simulink model "kalman"  (R2021a)
settings: Solver=VariableStepAuto  StartTime=0.0  StopTime=10.0  RelTol=1e-3
values from neighbouring files (symbols this model uses):
  A = [0,0,1,0;0,0,0,1;0,(g*mp)/mc,-d1/mc,-d2/(L*mc);0,(g*(mc+mp))/(L*mc),-d1/(L*mc),-(d2*(mc+mp))/(L*L*mc*mp)]    [assgn_4.m]
  B = [0;0;1/mc;1/(L*mc)]    [assgn_4.m]
  C = [1,0,0,0]    [assgn_4.m]
undefined symbols (not defined in the file or in its folder): K1
libraries: simulink x1
settings Model: Creator=hp  LastModifiedBy=hp

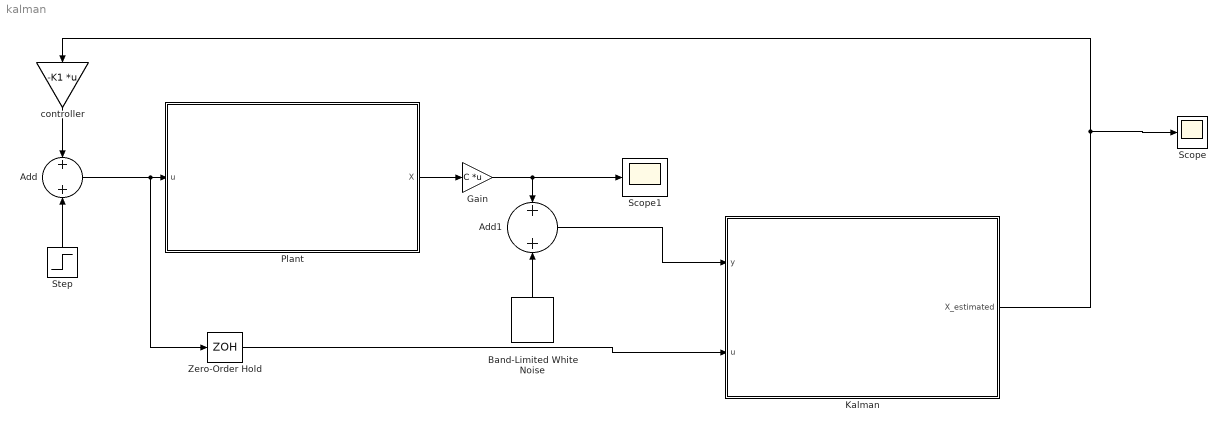
== system kalman ==
  Add : Sum
  Add1 : Sum
  Band-Limited White Noise : simulink/Sources/Band-Limited White Noise  Cov=[0.005]  Ts=0.1  seed=[23341]
  Gain : Gain  Gain=C  Multiplication=Matrix(K*u)
  Kalman : Subsystem
  Plant : Subsystem
  Scope : Scope
  Scope1 : Scope
  Step : Step  Time=0  SampleTime=0
  Zero-Order Hold : ZeroOrderHold  SampleTime=-1
  controller : Gain  Gain=-K1  Multiplication=Matrix(K*u)
  wires:
  Add/1 -> Plant/1(u), Zero-Order Hold/1
  Step/1 -> Add/2
  controller/1 -> Add/1
  Zero-Order Hold/1 -> Kalman/2(u)
  Plant/1(X) -> Gain/1
  Gain/1 -> Scope1/1, Add1/1
  Band-Limited White Noise/1 -> Add1/2
  Add1/1 -> Kalman/1(y)
  Kalman/1(X_estimated) -> Scope/1, controller/1

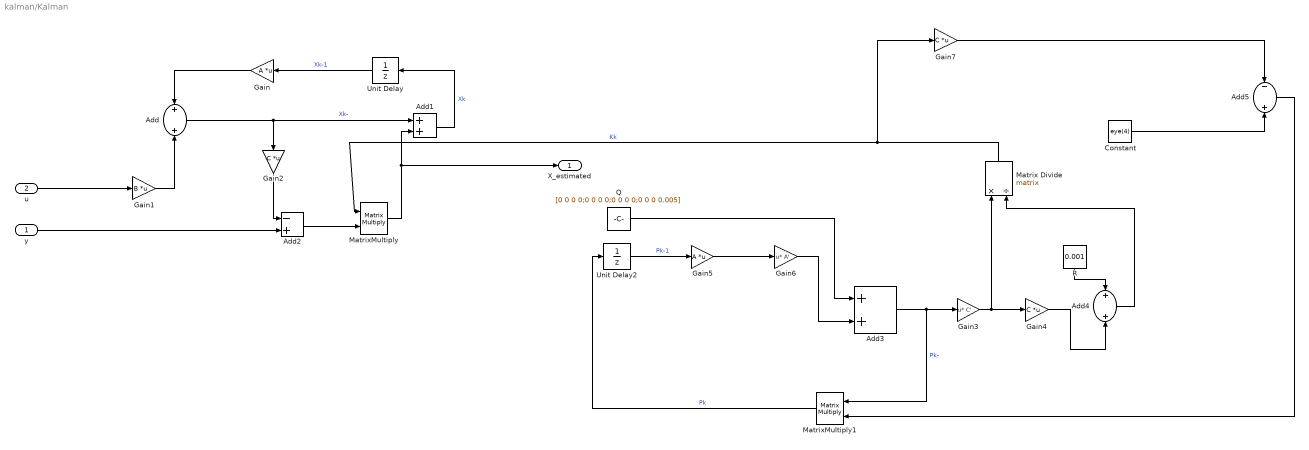
== system kalman/Kalman ==
  y : Inport
  u : Inport  Port=2
  Add{,1,3..4} (4 alike) : Sum
  Add2 : Sum  Inputs=-+
  Add5 : Sum  Inputs=-+
  Constant : Constant  Value=eye(4)
  Gain : Gain  Gain=A  Multiplication=Matrix(K*u)
  Gain1 : Gain  Gain=B  Multiplication=Matrix(K*u)
  Gain2 : Gain  Gain=C  Multiplication=Matrix(K*u)
  Gain3 : Gain  Gain=C'  Multiplication=Matrix(u*K)
  Gain4 : Gain  Gain=C  Multiplication=Matrix(K*u)
  Gain5 : Gain  Gain=A  Multiplication=Matrix(K*u)
  Gain6 : Gain  Gain=A'  Multiplication=Matrix(u*K)
  Gain7 : Gain  Gain=C  Multiplication=Matrix(K*u)
  Matrix Divide : Product  Inputs=*/  Multiplication=Matrix(*)
  MatrixMultiply : Product  Multiplication=Matrix(*)
  MatrixMultiply1 : Product  Multiplication=Matrix(*)
  Q : Constant  Value=[0 0 0 0;0 0 0 0;0 0 0 0;0 0 0 0.005]
  R : Constant  Value=0.001
  Unit Delay : UnitDelay  SampleTime=-1  HasFrameUpgradeWarning=on
  Unit Delay2 : UnitDelay  SampleTime=-1  HasFrameUpgradeWarning=on
  X_estimated : Outport
  wires:
  Gain/1 -> Add/1
  Unit Delay/1 -> Gain/1  "Xk-1"
  Gain2/1 -> Add2/1
  Add/1 -> Add1/1, Gain2/1  "Xk-"
  u/1 -> Gain1/1
  MatrixMultiply/1 -> Add1/2, X_estimated/1
  Add1/1 -> Unit Delay/1  "Xk"
  Gain1/1 -> Add/2
  y/1 -> Add2/2
  Add2/1 -> MatrixMultiply/2
  Matrix Divide/1 -> Gain7/1, MatrixMultiply/1  "Kk"
  MatrixMultiply1/1 -> Unit Delay2/1  "Pk"
  Gain6/1 -> Add3/2
  Gain5/1 -> Gain6/1
  Unit Delay2/1 -> Gain5/1  "Pk-1"
  Q/1 -> Add3/1
  Add3/1 -> MatrixMultiply1/1, Gain3/1  "Pk-"
  Gain3/1 -> Gain4/1, Matrix Divide/1
  Gain4/1 -> Add4/2
  R/1 -> Add4/1
  Add4/1 -> Matrix Divide/2
  Constant/1 -> Add5/2
  Gain7/1 -> Add5/1
  Add5/1 -> MatrixMultiply1/2

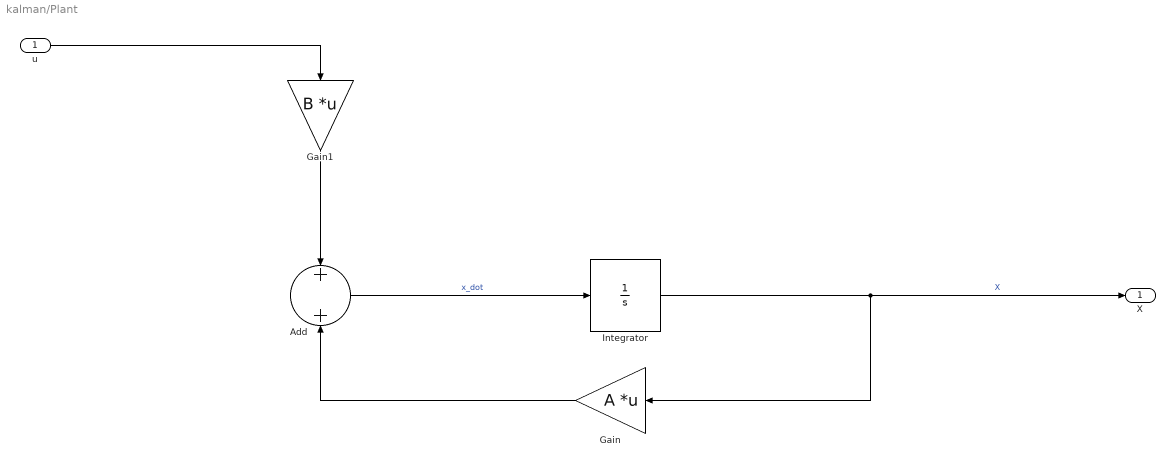
== system kalman/Plant ==
  u : Inport
  Add : Sum
  Gain : Gain  Gain=A  Multiplication=Matrix(K*u)
  Gain1 : Gain  Gain=B  Multiplication=Matrix(K*u)
  Integrator : Integrator  InitialCondition=0.17
  X : Outport
  wires:
  u/1 -> Gain1/1
  Gain1/1 -> Add/1
  Add/1 -> Integrator/1  "x_dot"
  Gain/1 -> Add/2
  Integrator/1 -> X/1, Gain/1  "X"
